simulink model "threephaserectifier"  (R2024b)
settings: Solver=VariableStepAuto  StartTime=0.0  StopTime=.1  RelTol=1e-3
libraries: spsThyristorLib x12, spsMonostableLib x6, simulink x6, spsSeriesRLCBranchLib x5, spsCurrentMeasurementLib x2, spsThreePhaseVIMeasurementLib x2, spsThreePhaseSourceLib x2, spsVoltageMeasurementLib x2, spspowerguiLib x1
settings Model: Creator=91798  LastModifiedBy=91798

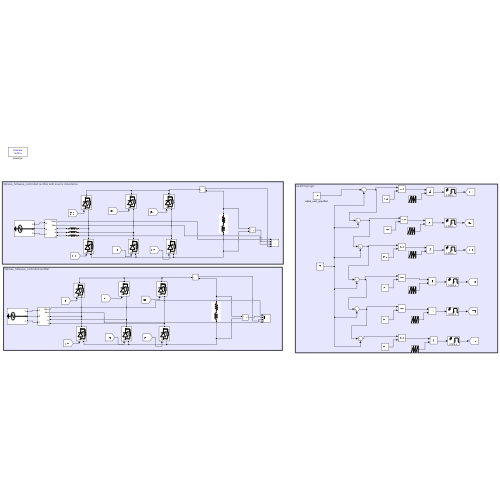
[thumbnail: Simulink's stored preview of the top-level diagram]
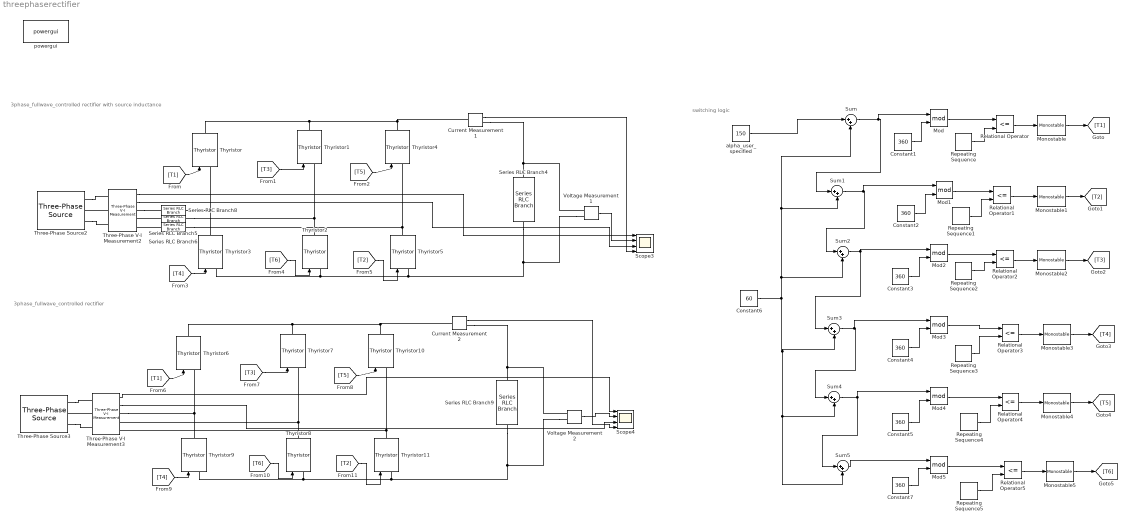
== system threephaserectifier ==
  note: switching logic
  note: 3phase_fullwave_controlled rectifier with source inductance
  note: 3phase_fullwave_controlled rectifier
  Constant{1..5,7} (6 alike) : Constant  Value=360
  Constant6 : Constant  Value=60
  Current Measurement1 : spsCurrentMeasurementLib/Current Measurement  PhasorSimulation=off  OutputType=Complex  PSBequivalent=0
  Current Measurement2 : spsCurrentMeasurementLib/Current Measurement  PhasorSimulation=off  OutputType=Complex  PSBequivalent=0
  Mod{,1..5} (6 alike) : Math  Operator=mod
  Monostable : spsMonostableLib/Monostable  EdgeDetect=Rising  PulseDuration=0.005  ic=0  Ts=0
      settings: LibrarySourceBlock=sps_lib/Control/Monostable
  Monostable1 : spsMonostableLib/Monostable  EdgeDetect=Rising  PulseDuration=0.005  ic=0  Ts=0
      settings: LibrarySourceBlock=sps_lib/Control/Monostable
  Monostable2 : spsMonostableLib/Monostable  EdgeDetect=Rising  PulseDuration=0.005  ic=0  Ts=0
      settings: LibrarySourceBlock=sps_lib/Control/Monostable
  Monostable3 : spsMonostableLib/Monostable  EdgeDetect=Rising  PulseDuration=0.004  ic=0  Ts=0
      settings: LibrarySourceBlock=sps_lib/Control/Monostable
  Monostable4 : spsMonostableLib/Monostable  EdgeDetect=Rising  PulseDuration=0.004  ic=0  Ts=0
      settings: LibrarySourceBlock=sps_lib/Control/Monostable
  Monostable5 : spsMonostableLib/Monostable  EdgeDetect=Rising  PulseDuration=0.004  ic=0  Ts=0
      settings: LibrarySourceBlock=sps_lib/Control/Monostable
  Relational Operator{,1..5} (6 alike) : RelationalOperator  Operator=<=  OutDataTypeStr=boolean  RndMeth=Simplest  InputSameDT=off
  Repeating Sequence{,1..2,4..5} (5 alike) : simulink/Sources/Repeating Sequence  rep_seq_t=[0 0.02]  rep_seq_y=[0 360]
  Repeating Sequence3 : simulink/Sources/Repeating Sequence  rep_seq_t=[0 0.02]  rep_seq_y=[0 360.1]
  Scope3 : Scope  NumInputPorts=4
  Scope4 : Scope  NumInputPorts=4
  Series RLC Branch4 : spsSeriesRLCBranchLib/Series RLC Branch  LConnTagsString=__new0  RConnTagsString=__new0  BranchType=RL  Resistance=20  Inductance=20e-3  SetiL0=off  InitialCurrent=0  Capacitance=1e-6  Setx0=off  InitialVoltage=0  Measurements=None
  Series RLC Branch5 : spsSeriesRLCBranchLib/Series RLC Branch  LConnTagsString=__new0  RConnTagsString=__new0  BranchType=L  Resistance=10e-3  Inductance=10e-3  SetiL0=off  InitialCurrent=0  Capacitance=1e-6  Setx0=off  InitialVoltage=0  Measurements=None
  Series RLC Branch6 : spsSeriesRLCBranchLib/Series RLC Branch  LConnTagsString=__new0  RConnTagsString=__new0  BranchType=L  Resistance=10e-3  Inductance=10e-3  SetiL0=off  InitialCurrent=0  Capacitance=1e-6  Setx0=off  InitialVoltage=0  Measurements=None
  Series RLC Branch8 : spsSeriesRLCBranchLib/Series RLC Branch  LConnTagsString=__new0  RConnTagsString=__new0  BranchType=L  Resistance=10e-3  Inductance=10e-3  SetiL0=off  InitialCurrent=0  Capacitance=1e-6  Setx0=off  InitialVoltage=0  Measurements=None
  Series RLC Branch9 : spsSeriesRLCBranchLib/Series RLC Branch  LConnTagsString=__new0  RConnTagsString=__new0  BranchType=RL  Resistance=20  Inductance=20e-3  SetiL0=off  InitialCurrent=0  Capacitance=1e-6  Setx0=off  InitialVoltage=0  Measurements=None
  Sum{,1..5} (6 alike) : Sum  Inputs=|++
  Three-Phase V-I Measurement2 : spsThreePhaseVIMeasurementLib/Three-Phase V-I Measurement  VoltageMeasurement=phase-to-phase  SetLabelV=off  LabelV=Vabc  Vpu=off  VpuLL=off  CurrentMeasurement=yes  SetLabelI=off  LabelI=Iabc  Ipu=off  Pbase=100e6  Vbase=500e3  OutputType=Complex  PhasorSimulation=off  PSBequivalent=0
  Three-Phase V-I Measurement3 : spsThreePhaseVIMeasurementLib/Three-Phase V-I Measurement  VoltageMeasurement=phase-to-phase  SetLabelV=off  LabelV=Vabc  Vpu=off  VpuLL=off  CurrentMeasurement=yes  SetLabelI=off  LabelI=Iabc  Ipu=off  Pbase=100e6  Vbase=500e3  OutputType=Complex  PhasorSimulation=off  PSBequivalent=0
  Three-Phase Source2 : spsThreePhaseSourceLib/Three-Phase Source  InternalConnection=Yg  VoltagePhases=off  Voltage=400  PhaseAngle=0  Voltage_phases=[25e3 25e3 25e3]/sqrt(3)  PhaseAngles_phases=[0 -120 +120]  Frequency=50  NonIdealSource=off  SpecifyImpedance=off  Resistance=0  Inductance=10e-3  ShortCircuitLevel=100e6  BaseVoltage=2500  XRratio=7  BusType=swing  Pref=10e3  Qref=0  Prefabc=[10e3, 10e3, 10e3]  Qrefabc=[0, 0, 0]  Qmin=-inf  Qmax=inf
  Three-Phase Source3 : spsThreePhaseSourceLib/Three-Phase Source  InternalConnection=Yg  VoltagePhases=off  Voltage=400  PhaseAngle=0  Voltage_phases=[25e3 25e3 25e3]/sqrt(3)  PhaseAngles_phases=[0 -120 +120]  Frequency=50  NonIdealSource=off  SpecifyImpedance=off  Resistance=0  Inductance=10e-3  ShortCircuitLevel=100e6  BaseVoltage=2500  XRratio=7  BusType=swing  Pref=10e3  Qref=0  Prefabc=[10e3, 10e3, 10e3]  Qrefabc=[0, 0, 0]  Qmin=-inf  Qmax=inf
  Thyristor{,1..11} (12 alike) : spsThyristorLib/Thyristor  Ron=0.001  Lon=0  Vf=0.8  IC=0  Rs=500  Cs=250e-9  Measurements=off
  Voltage Measurement1 : spsVoltageMeasurementLib/Voltage Measurement  PhasorSimulation=off  OutputType=Complex  PSBequivalent=0
  Voltage Measurement2 : spsVoltageMeasurementLib/Voltage Measurement  PhasorSimulation=off  OutputType=Complex  PSBequivalent=0
  alpha_user_specified : Constant  Value=150
  powergui : spspowerguiLib/powergui  Priority=1  SimulationMode=Discrete  SampleTime=1e-6  frequency=60  Iterations=50  frequencyindice=0  Pbase=100e6  ErrMax=1e-4  UnitsV=kV  UnitsW=MW  buscounter=0  FunctionMessages=off  echomessages=off  EnableUseOfTLC=off  CurrentSourceSwitches=off  DisableSnubberDevices=off  DisableRonSwitches=off  DisableVfSwitches=off  DisplayEquations=off  AutomaticDiscreteSolvers=off  SolverType=Tustin/Backward Euler (TBE)  Interpol=off  ExternalGateDelay=off  methode=off  Ts=100  x0status=blocks  SPID=on  SwTol=0  HookPort=off  NonlinearTolerance=1e-4  nMaxIteration=100  ContinueOnMaxIteration=off  RestoreLinks=warning  ResistiveCurrentMeasurement=off  Frange=[0:2:500]  Ylog=off  Xlog=on  ShowGrid=off  save=off  variable=ZData  structure=0  ZoomFFT=off  StartTime=0.0  cycles=1  DisplayStyle=1  fundamental=60  FreqAxis=off  MaxFrequency=1000  frequencyindicesteady=1  RmsSteady=1  display=off
  wires:
  Relational Operator/1 -> Monostable/1
  [T4] -> Thyristor3/1
  Monostable5/1 -> [T6]
  Three-Phase V-I Measurement2/2 -> Scope3/3
  Relational Operator2/1 -> Monostable2/1
  [T6] -> Thyristor2/1
  Sum4/1 -> Mod4/1, Sum5/1
  Sum3/1 -> Mod3/1, Sum4/1
  [T2] -> Thyristor5/1
  Sum/1 -> Mod/1, Sum1/1
  Voltage Measurement1/1 -> Scope3/2
  Relational Operator3/1 -> Monostable3/1
  Current Measurement1/1 -> Scope3/4
  Repeating Sequence3/1 -> Relational Operator3/2
  Repeating Sequence2/1 -> Relational Operator2/2
  Monostable/1 -> [T1]
  Relational Operator4/1 -> Monostable4/1
  [T1] -> Thyristor/1
  [T5] -> Thyristor4/1
  Repeating Sequence5/1 -> Relational Operator5/2
  Repeating Sequence4/1 -> Relational Operator4/2
  Monostable4/1 -> [T5]
  Monostable3/1 -> [T4]
  Sum2/1 -> Mod2/1, Sum3/1
  Three-Phase V-I Measurement2/1 -> Scope3/1
  [T3] -> Thyristor1/1
  Relational Operator5/1 -> Monostable5/1
  Repeating Sequence/1 -> Relational Operator/2
  Monostable2/1 -> [T3]
  alpha_user_specified/1 -> Sum/1
  Constant6/1 -> Sum1/2, Sum/2, Sum2/2, Sum3/2, Sum5/2, Sum4/2
  Sum1/1 -> Mod1/1, Sum2/1
  Repeating Sequence1/1 -> Relational Operator1/2
  Monostable1/1 -> [T2]
  Relational Operator1/1 -> Monostable1/1
  [T4] -> Thyristor9/1
  [T3] -> Thyristor7/1
  [T1] -> Thyristor6/1
  [T2] -> Thyristor11/1
  [T6] -> Thyristor8/1
  Current Measurement2/1 -> Scope4/4
  Three-Phase V-I Measurement3/1 -> Scope4/1
  Voltage Measurement2/1 -> Scope4/2
  Three-Phase V-I Measurement3/2 -> Scope4/3
  [T5] -> Thyristor10/1
  Constant1/1 -> Mod/2
  Constant2/1 -> Mod1/2
  Mod1/1 -> Relational Operator1/1
  Mod/1 -> Relational Operator/1
  Constant3/1 -> Mod2/2
  Mod2/1 -> Relational Operator2/1
  Constant4/1 -> Mod3/2
  Mod3/1 -> Relational Operator3/1
  Constant5/1 -> Mod4/2
  Mod4/1 -> Relational Operator4/1
  Constant7/1 -> Mod5/2
  Mod5/1 -> Relational Operator5/1
  Sum5/1 -> Mod5/1
  connections:
  Thyristor4/LConn1 -- Thyristor5/RConn1 -- Series RLC Branch6/LConn1
  Thyristor/LConn1 -- Thyristor3/RConn1 -- Series RLC Branch8/LConn1
  Thyristor1/LConn1 -- Thyristor2/RConn1 -- Series RLC Branch5/LConn1
  Voltage Measurement1/LConn2 -- Thyristor2/LConn1 -- Thyristor3/LConn1 -- Thyristor5/LConn1 -- Series RLC Branch4/RConn1
  Thyristor4/RConn1 -- Thyristor/RConn1 -- Thyristor1/RConn1 -- Current Measurement1/LConn1
  Voltage Measurement1/LConn1 -- Series RLC Branch4/LConn1 -- Current Measurement1/RConn1
  Series RLC Branch5/RConn1 -- Three-Phase V-I Measurement2/RConn2
  Three-Phase Source2/RConn3 -- Three-Phase V-I Measurement2/LConn3
  Three-Phase V-I Measurement2/LConn2 -- Three-Phase Source2/RConn2
  Three-Phase Source2/RConn1 -- Three-Phase V-I Measurement2/LConn1
  Three-Phase V-I Measurement2/RConn1 -- Series RLC Branch8/RConn1
  Series RLC Branch6/RConn1 -- Three-Phase V-I Measurement2/RConn3
  Voltage Measurement2/LConn2 -- Thyristor8/LConn1 -- Thyristor9/LConn1 -- Thyristor11/LConn1 -- Series RLC Branch9/RConn1
  Voltage Measurement2/LConn1 -- Series RLC Branch9/LConn1 -- Current Measurement2/RConn1
  Thyristor10/RConn1 -- Thyristor6/RConn1 -- Thyristor7/RConn1 -- Current Measurement2/LConn1
  Three-Phase Source3/RConn3 -- Three-Phase V-I Measurement3/LConn3
  Three-Phase Source3/RConn1 -- Three-Phase V-I Measurement3/LConn1
  Thyristor7/LConn1 -- Thyristor8/RConn1 -- Three-Phase V-I Measurement3/RConn2
  Three-Phase V-I Measurement3/LConn2 -- Three-Phase Source3/RConn2
  Thyristor6/LConn1 -- Three-Phase V-I Measurement3/RConn1 -- Thyristor9/RConn1
  Thyristor10/LConn1 -- Three-Phase V-I Measurement3/RConn3 -- Thyristor11/RConn1
